simulink model "aileronAssembly"  (R2025a)
settings: Solver=VariableStepAuto  StartTime=0.0  StopTime=10.0  RelTol=1e-3
model workspace: external: MATLAB File aileronAssembly_DataFile.m (data not in the file)
undefined symbols (not defined in the file or in its folder): smiData, X, Y, Z
libraries: sm_lib x604, nesl_utility x1
(part 2 of 10)

== system aileronAssembly/Actuator_3/Cylinder_1_RIGID ==
  ReferenceFrame : sm_lib/Frames and Transforms/Reference Frame
  Solid : sm_lib/Body Elements/File Solid  ExtGeomFileName=Cylinder.step  UnitType=FromFile  ExtGeomFileUnits=m  StepReaderType=HEX  ExportConvexHullGeometry=off  InertiaType=Custom  BasedOnType=Density  Density=1000  DensityUnits=kg/m^3  Mass=smiData.Solid(7).mass  MassUnits=kg  CenterOfMass=smiData.Solid(7).CoM  CenterOfMassUnits=m  MomentsOfInertia=smiData.Solid(7).MoI  MomentsOfInertiaUnits=kg*m^2  ProductsOfInertia=smiData.Solid(7).PoI  ProductsOfInertiaUnits=kg*m^2  GraphicType=FromGeometry  MarkerShape=Sphere  MarkerSize=10  GraphicVisPropType=SimpleVisualProperties  GraphicDiffuseColor=smiData.Solid(7).color  GraphicOpacity=smiData.Solid(7).opacity  GraphicSpecularColor=[0.5 0.5 0.5 1.0]  GraphicAmbientColor=[0.15 0.15 0.15 1.0]  GraphicEmissiveColor=[0.0 0.0 0.0 1.0]  GraphicShininess=75  DoExposeReferenceFrame=on  SerializedFrames=<Frames/>
  Transform : sm_lib/Frames and Transforms/Rigid Transform  RotationMethod=ArbitraryAxis  FollAlignAxisA=+X  BaseAlignAxisA=+Y  FollAlignAxisB=+Y  BaseAlignAxisB=+Z  RotationStandardAxis=+Z  RotationAngle=smiData.RigidTransform(169).angle  RotationAngleUnits=rad  RotationArbitraryAxis=smiData.RigidTransform(169).axis  RotationSequenceAxes=FollowerAxes  RotationSequence=XYX  RotationSequenceAngles=[0 0 0]  RotationSequenceAnglesUnits=deg  RotationMatrix=[1 0 0; 0 1 0; 0 0 1]  Quaternion=[1 0 0 0]  TranslationMethod=Cartesian  TranslationCartesianOffset=smiData.RigidTransform(169).translation  TranslationCartesianOffsetUnits=m  TranslationStandardAxis=+Z  TranslationStandardOffset=0  TranslationStandardOffsetUnits=m  TranslationROffset=0  TranslationROffsetUnits=m  TranslationThetaOffset=0  TranslationThetaOffsetUnits=deg  TranslationZOffset=0  TranslationZOffsetUnits=m
  Transform1 : sm_lib/Frames and Transforms/Rigid Transform  RotationMethod=ArbitraryAxis  FollAlignAxisA=+X  BaseAlignAxisA=+Y  FollAlignAxisB=+Y  BaseAlignAxisB=+Z  RotationStandardAxis=+Z  RotationAngle=smiData.RigidTransform(196).angle  RotationAngleUnits=rad  RotationArbitraryAxis=smiData.RigidTransform(196).axis  RotationSequenceAxes=FollowerAxes  RotationSequence=XYX  RotationSequenceAngles=[0 0 0]  RotationSequenceAnglesUnits=deg  RotationMatrix=[1 0 0; 0 1 0; 0 0 1]  Quaternion=[1 0 0 0]  TranslationMethod=Cartesian  TranslationCartesianOffset=smiData.RigidTransform(196).translation  TranslationCartesianOffsetUnits=m  TranslationStandardAxis=+Z  TranslationStandardOffset=0  TranslationStandardOffsetUnits=m  TranslationROffset=0  TranslationROffsetUnits=m  TranslationThetaOffset=0  TranslationThetaOffsetUnits=deg  TranslationZOffset=0  TranslationZOffsetUnits=m
  F1 : PMIOPort  Side=Left
  F : PMIOPort  Port=2  Side=Right
  connections:
  Solid/RConn1 -- ReferenceFrame/RConn1 -- Transform/LConn1 -- Transform1/LConn1
  Transform/RConn1 -- F/RConn1
  Transform1/RConn1 -- F1/RConn1

== system aileronAssembly/Actuator_3/Piston_1_RIGID ==
  ReferenceFrame : sm_lib/Frames and Transforms/Reference Frame
  Solid : sm_lib/Body Elements/File Solid  ExtGeomFileName=Piston.step  UnitType=FromFile  ExtGeomFileUnits=m  StepReaderType=HEX  ExportConvexHullGeometry=off  InertiaType=Custom  BasedOnType=Density  Density=1000  DensityUnits=kg/m^3  Mass=smiData.Solid(8).mass  MassUnits=kg  CenterOfMass=smiData.Solid(8).CoM  CenterOfMassUnits=m  MomentsOfInertia=smiData.Solid(8).MoI  MomentsOfInertiaUnits=kg*m^2  ProductsOfInertia=smiData.Solid(8).PoI  ProductsOfInertiaUnits=kg*m^2  GraphicType=FromGeometry  MarkerShape=Sphere  MarkerSize=10  GraphicVisPropType=SimpleVisualProperties  GraphicDiffuseColor=smiData.Solid(8).color  GraphicOpacity=smiData.Solid(8).opacity  GraphicSpecularColor=[0.5 0.5 0.5 1.0]  GraphicAmbientColor=[0.15 0.15 0.15 1.0]  GraphicEmissiveColor=[0.0 0.0 0.0 1.0]  GraphicShininess=75  DoExposeReferenceFrame=on  SerializedFrames=<Frames/>
  Transform : sm_lib/Frames and Transforms/Rigid Transform  RotationMethod=ArbitraryAxis  FollAlignAxisA=+X  BaseAlignAxisA=+Y  FollAlignAxisB=+Y  BaseAlignAxisB=+Z  RotationStandardAxis=+Z  RotationAngle=smiData.RigidTransform(170).angle  RotationAngleUnits=rad  RotationArbitraryAxis=smiData.RigidTransform(170).axis  RotationSequenceAxes=FollowerAxes  RotationSequence=XYX  RotationSequenceAngles=[0 0 0]  RotationSequenceAnglesUnits=deg  RotationMatrix=[1 0 0; 0 1 0; 0 0 1]  Quaternion=[1 0 0 0]  TranslationMethod=Cartesian  TranslationCartesianOffset=smiData.RigidTransform(170).translation  TranslationCartesianOffsetUnits=m  TranslationStandardAxis=+Z  TranslationStandardOffset=0  TranslationStandardOffsetUnits=m  TranslationROffset=0  TranslationROffsetUnits=m  TranslationThetaOffset=0  TranslationThetaOffsetUnits=deg  TranslationZOffset=0  TranslationZOffsetUnits=m
  Transform1 : sm_lib/Frames and Transforms/Rigid Transform  RotationMethod=ArbitraryAxis  FollAlignAxisA=+X  BaseAlignAxisA=+Y  FollAlignAxisB=+Y  BaseAlignAxisB=+Z  RotationStandardAxis=+Z  RotationAngle=smiData.RigidTransform(201).angle  RotationAngleUnits=rad  RotationArbitraryAxis=smiData.RigidTransform(201).axis  RotationSequenceAxes=FollowerAxes  RotationSequence=XYX  RotationSequenceAngles=[0 0 0]  RotationSequenceAnglesUnits=deg  RotationMatrix=[1 0 0; 0 1 0; 0 0 1]  Quaternion=[1 0 0 0]  TranslationMethod=Cartesian  TranslationCartesianOffset=smiData.RigidTransform(201).translation  TranslationCartesianOffsetUnits=m  TranslationStandardAxis=+Z  TranslationStandardOffset=0  TranslationStandardOffsetUnits=m  TranslationROffset=0  TranslationROffsetUnits=m  TranslationThetaOffset=0  TranslationThetaOffsetUnits=deg  TranslationZOffset=0  TranslationZOffsetUnits=m
  F1 : PMIOPort  Side=Left
  F : PMIOPort  Port=2  Side=Left
  connections:
  Solid/RConn1 -- ReferenceFrame/RConn1 -- Transform/LConn1 -- Transform1/LConn1
  Transform/RConn1 -- F/RConn1
  Transform1/RConn1 -- F1/RConn1

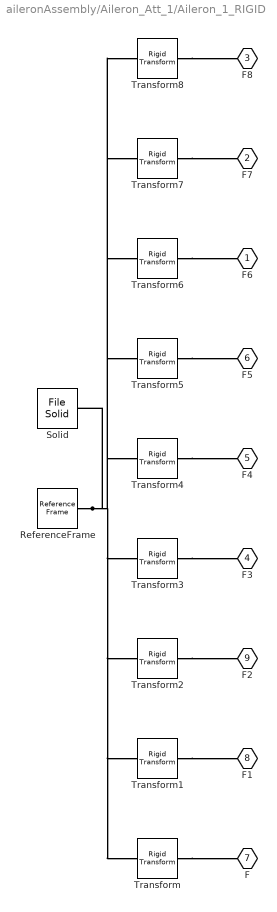
== system aileronAssembly/Aileron_Att_1/Aileron_1_RIGID ==
  ReferenceFrame : sm_lib/Frames and Transforms/Reference Frame
  Solid : sm_lib/Body Elements/File Solid  ExtGeomFileName=Aileron.step  UnitType=FromFile  ExtGeomFileUnits=m  StepReaderType=HEX  ExportConvexHullGeometry=off  InertiaType=Custom  BasedOnType=Density  Density=1000  DensityUnits=kg/m^3  Mass=smiData.Solid(9).mass  MassUnits=kg  CenterOfMass=smiData.Solid(9).CoM  CenterOfMassUnits=m  MomentsOfInertia=smiData.Solid(9).MoI  MomentsOfInertiaUnits=kg*m^2  ProductsOfInertia=smiData.Solid(9).PoI  ProductsOfInertiaUnits=kg*m^2  GraphicType=FromGeometry  MarkerShape=Sphere  MarkerSize=10  GraphicVisPropType=SimpleVisualProperties  GraphicDiffuseColor=smiData.Solid(9).color  GraphicOpacity=smiData.Solid(9).opacity  GraphicSpecularColor=[0.5 0.5 0.5 1.0]  GraphicAmbientColor=[0.15 0.15 0.15 1.0]  GraphicEmissiveColor=[0.0 0.0 0.0 1.0]  GraphicShininess=75  DoExposeReferenceFrame=on  SerializedFrames=<Frames/>
  Transform : sm_lib/Frames and Transforms/Rigid Transform  RotationMethod=ArbitraryAxis  FollAlignAxisA=+X  BaseAlignAxisA=+Y  FollAlignAxisB=+Y  BaseAlignAxisB=+Z  RotationStandardAxis=+Z  RotationAngle=smiData.RigidTransform(171).angle  RotationAngleUnits=rad  RotationArbitraryAxis=smiData.RigidTransform(171).axis  RotationSequenceAxes=FollowerAxes  RotationSequence=XYX  RotationSequenceAngles=[0 0 0]  RotationSequenceAnglesUnits=deg  RotationMatrix=[1 0 0; 0 1 0; 0 0 1]  Quaternion=[1 0 0 0]  TranslationMethod=Cartesian  TranslationCartesianOffset=smiData.RigidTransform(171).translation  TranslationCartesianOffsetUnits=m  TranslationStandardAxis=+Z  TranslationStandardOffset=0  TranslationStandardOffsetUnits=m  TranslationROffset=0  TranslationROffsetUnits=m  TranslationThetaOffset=0  TranslationThetaOffsetUnits=deg  TranslationZOffset=0  TranslationZOffsetUnits=m
  Transform1 : sm_lib/Frames and Transforms/Rigid Transform  RotationMethod=ArbitraryAxis  FollAlignAxisA=+X  BaseAlignAxisA=+Y  FollAlignAxisB=+Y  BaseAlignAxisB=+Z  RotationStandardAxis=+Z  RotationAngle=smiData.RigidTransform(173).angle  RotationAngleUnits=rad  RotationArbitraryAxis=smiData.RigidTransform(173).axis  RotationSequenceAxes=FollowerAxes  RotationSequence=XYX  RotationSequenceAngles=[0 0 0]  RotationSequenceAnglesUnits=deg  RotationMatrix=[1 0 0; 0 1 0; 0 0 1]  Quaternion=[1 0 0 0]  TranslationMethod=Cartesian  TranslationCartesianOffset=smiData.RigidTransform(173).translation  TranslationCartesianOffsetUnits=m  TranslationStandardAxis=+Z  TranslationStandardOffset=0  TranslationStandardOffsetUnits=m  TranslationROffset=0  TranslationROffsetUnits=m  TranslationThetaOffset=0  TranslationThetaOffsetUnits=deg  TranslationZOffset=0  TranslationZOffsetUnits=m
  Transform2 : sm_lib/Frames and Transforms/Rigid Transform  RotationMethod=ArbitraryAxis  FollAlignAxisA=+X  BaseAlignAxisA=+Y  FollAlignAxisB=+Y  BaseAlignAxisB=+Z  RotationStandardAxis=+Z  RotationAngle=smiData.RigidTransform(175).angle  RotationAngleUnits=rad  RotationArbitraryAxis=smiData.RigidTransform(175).axis  RotationSequenceAxes=FollowerAxes  RotationSequence=XYX  RotationSequenceAngles=[0 0 0]  RotationSequenceAnglesUnits=deg  RotationMatrix=[1 0 0; 0 1 0; 0 0 1]  Quaternion=[1 0 0 0]  TranslationMethod=Cartesian  TranslationCartesianOffset=smiData.RigidTransform(175).translation  TranslationCartesianOffsetUnits=m  TranslationStandardAxis=+Z  TranslationStandardOffset=0  TranslationStandardOffsetUnits=m  TranslationROffset=0  TranslationROffsetUnits=m  TranslationThetaOffset=0  TranslationThetaOffsetUnits=deg  TranslationZOffset=0  TranslationZOffsetUnits=m
  Transform3 : sm_lib/Frames and Transforms/Rigid Transform  RotationMethod=ArbitraryAxis  FollAlignAxisA=+X  BaseAlignAxisA=+Y  FollAlignAxisB=+Y  BaseAlignAxisB=+Z  RotationStandardAxis=+Z  RotationAngle=smiData.RigidTransform(177).angle  RotationAngleUnits=rad  RotationArbitraryAxis=smiData.RigidTransform(177).axis  RotationSequenceAxes=FollowerAxes  RotationSequence=XYX  RotationSequenceAngles=[0 0 0]  RotationSequenceAnglesUnits=deg  RotationMatrix=[1 0 0; 0 1 0; 0 0 1]  Quaternion=[1 0 0 0]  TranslationMethod=Cartesian  TranslationCartesianOffset=smiData.RigidTransform(177).translation  TranslationCartesianOffsetUnits=m  TranslationStandardAxis=+Z  TranslationStandardOffset=0  TranslationStandardOffsetUnits=m  TranslationROffset=0  TranslationROffsetUnits=m  TranslationThetaOffset=0  TranslationThetaOffsetUnits=deg  TranslationZOffset=0  TranslationZOffsetUnits=m
  Transform4 : sm_lib/Frames and Transforms/Rigid Transform  RotationMethod=ArbitraryAxis  FollAlignAxisA=+X  BaseAlignAxisA=+Y  FollAlignAxisB=+Y  BaseAlignAxisB=+Z  RotationStandardAxis=+Z  RotationAngle=smiData.RigidTransform(180).angle  RotationAngleUnits=rad  RotationArbitraryAxis=smiData.RigidTransform(180).axis  RotationSequenceAxes=FollowerAxes  RotationSequence=XYX  RotationSequenceAngles=[0 0 0]  RotationSequenceAnglesUnits=deg  RotationMatrix=[1 0 0; 0 1 0; 0 0 1]  Quaternion=[1 0 0 0]  TranslationMethod=Cartesian  TranslationCartesianOffset=smiData.RigidTransform(180).translation  TranslationCartesianOffsetUnits=m  TranslationStandardAxis=+Z  TranslationStandardOffset=0  TranslationStandardOffsetUnits=m  TranslationROffset=0  TranslationROffsetUnits=m  TranslationThetaOffset=0  TranslationThetaOffsetUnits=deg  TranslationZOffset=0  TranslationZOffsetUnits=m
  Transform5 : sm_lib/Frames and Transforms/Rigid Transform  RotationMethod=ArbitraryAxis  FollAlignAxisA=+X  BaseAlignAxisA=+Y  FollAlignAxisB=+Y  BaseAlignAxisB=+Z  RotationStandardAxis=+Z  RotationAngle=smiData.RigidTransform(182).angle  RotationAngleUnits=rad  RotationArbitraryAxis=smiData.RigidTransform(182).axis  RotationSequenceAxes=FollowerAxes  RotationSequence=XYX  RotationSequenceAngles=[0 0 0]  RotationSequenceAnglesUnits=deg  RotationMatrix=[1 0 0; 0 1 0; 0 0 1]  Quaternion=[1 0 0 0]  TranslationMethod=Cartesian  TranslationCartesianOffset=smiData.RigidTransform(182).translation  TranslationCartesianOffsetUnits=m  TranslationStandardAxis=+Z  TranslationStandardOffset=0  TranslationStandardOffsetUnits=m  TranslationROffset=0  TranslationROffsetUnits=m  TranslationThetaOffset=0  TranslationThetaOffsetUnits=deg  TranslationZOffset=0  TranslationZOffsetUnits=m
  Transform6 : sm_lib/Frames and Transforms/Rigid Transform  RotationMethod=ArbitraryAxis  FollAlignAxisA=+X  BaseAlignAxisA=+Y  FollAlignAxisB=+Y  BaseAlignAxisB=+Z  RotationStandardAxis=+Z  RotationAngle=smiData.RigidTransform(184).angle  RotationAngleUnits=rad  RotationArbitraryAxis=smiData.RigidTransform(184).axis  RotationSequenceAxes=FollowerAxes  RotationSequence=XYX  RotationSequenceAngles=[0 0 0]  RotationSequenceAnglesUnits=deg  RotationMatrix=[1 0 0; 0 1 0; 0 0 1]  Quaternion=[1 0 0 0]  TranslationMethod=Cartesian  TranslationCartesianOffset=smiData.RigidTransform(184).translation  TranslationCartesianOffsetUnits=m  TranslationStandardAxis=+Z  TranslationStandardOffset=0  TranslationStandardOffsetUnits=m  TranslationROffset=0  TranslationROffsetUnits=m  TranslationThetaOffset=0  TranslationThetaOffsetUnits=deg  TranslationZOffset=0  TranslationZOffsetUnits=m
  Transform7 : sm_lib/Frames and Transforms/Rigid Transform  RotationMethod=ArbitraryAxis  FollAlignAxisA=+X  BaseAlignAxisA=+Y  FollAlignAxisB=+Y  BaseAlignAxisB=+Z  RotationStandardAxis=+Z  RotationAngle=smiData.RigidTransform(186).angle  RotationAngleUnits=rad  RotationArbitraryAxis=smiData.RigidTransform(186).axis  RotationSequenceAxes=FollowerAxes  RotationSequence=XYX  RotationSequenceAngles=[0 0 0]  RotationSequenceAnglesUnits=deg  RotationMatrix=[1 0 0; 0 1 0; 0 0 1]  Quaternion=[1 0 0 0]  TranslationMethod=Cartesian  TranslationCartesianOffset=smiData.RigidTransform(186).translation  TranslationCartesianOffsetUnits=m  TranslationStandardAxis=+Z  TranslationStandardOffset=0  TranslationStandardOffsetUnits=m  TranslationROffset=0  TranslationROffsetUnits=m  TranslationThetaOffset=0  TranslationThetaOffsetUnits=deg  TranslationZOffset=0  TranslationZOffsetUnits=m
  Transform8 : sm_lib/Frames and Transforms/Rigid Transform  RotationMethod=ArbitraryAxis  FollAlignAxisA=+X  BaseAlignAxisA=+Y  FollAlignAxisB=+Y  BaseAlignAxisB=+Z  RotationStandardAxis=+Z  RotationAngle=smiData.RigidTransform(188).angle  RotationAngleUnits=rad  RotationArbitraryAxis=smiData.RigidTransform(188).axis  RotationSequenceAxes=FollowerAxes  RotationSequence=XYX  RotationSequenceAngles=[0 0 0]  RotationSequenceAnglesUnits=deg  RotationMatrix=[1 0 0; 0 1 0; 0 0 1]  Quaternion=[1 0 0 0]  TranslationMethod=Cartesian  TranslationCartesianOffset=smiData.RigidTransform(188).translation  TranslationCartesianOffsetUnits=m  TranslationStandardAxis=+Z  TranslationStandardOffset=0  TranslationStandardOffsetUnits=m  TranslationROffset=0  TranslationROffsetUnits=m  TranslationThetaOffset=0  TranslationThetaOffsetUnits=deg  TranslationZOffset=0  TranslationZOffsetUnits=m
  F6 : PMIOPort  Side=Left
  F7 : PMIOPort  Port=2  Side=Left
  F8 : PMIOPort  Port=3  Side=Left
  F3 : PMIOPort  Port=4  Side=Left
  F4 : PMIOPort  Port=5  Side=Left
  F5 : PMIOPort  Port=6  Side=Left
  F : PMIOPort  Port=7  Side=Left
  F1 : PMIOPort  Port=8  Side=Left
  F2 : PMIOPort  Port=9  Side=Left
  connections:
  Solid/RConn1 -- ReferenceFrame/RConn1 -- Transform/LConn1 -- Transform1/LConn1 -- Transform2/LConn1 -- Transform3/LConn1 -- Transform4/LConn1 -- Transform5/LConn1 -- Transform6/LConn1 -- Transform7/LConn1 -- Transform8/LConn1
  Transform/RConn1 -- F/RConn1
  Transform1/RConn1 -- F1/RConn1
  Transform2/RConn1 -- F2/RConn1
  Transform3/RConn1 -- F3/RConn1
  Transform4/RConn1 -- F4/RConn1
  Transform5/RConn1 -- F5/RConn1
  Transform6/RConn1 -- F6/RConn1
  Transform7/RConn1 -- F7/RConn1
  Transform8/RConn1 -- F8/RConn1

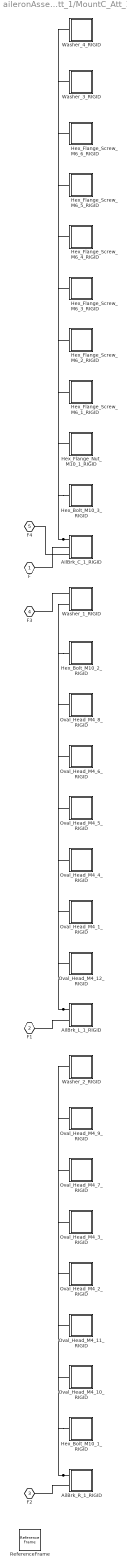
== system aileronAssembly/Aileron_Att_1/MountC_Att_1 ==
  AilBrk_C_1_RIGID : Subsystem
  AilBrk_L_1_RIGID : Subsystem
  AilBrk_R_1_RIGID : Subsystem
  Hex_Bolt_M10_1_RIGID : Subsystem
  Hex_Bolt_M10_2_RIGID : Subsystem
  Hex_Bolt_M10_3_RIGID : Subsystem
  Hex_Flange_Nut_M10_1_RIGID : Subsystem
  Hex_Flange_Screw_M6_1_RIGID : Subsystem
  Hex_Flange_Screw_M6_2_RIGID : Subsystem
  Hex_Flange_Screw_M6_3_RIGID : Subsystem
  Hex_Flange_Screw_M6_4_RIGID : Subsystem
  Hex_Flange_Screw_M6_5_RIGID : Subsystem
  Hex_Flange_Screw_M6_6_RIGID : Subsystem
  Oval_Head_M4_10_RIGID : Subsystem
  Oval_Head_M4_11_RIGID : Subsystem
  Oval_Head_M4_12_RIGID : Subsystem
  Oval_Head_M4_1_RIGID : Subsystem
  Oval_Head_M4_2_RIGID : Subsystem
  Oval_Head_M4_3_RIGID : Subsystem
  Oval_Head_M4_4_RIGID : Subsystem
  Oval_Head_M4_5_RIGID : Subsystem
  Oval_Head_M4_6_RIGID : Subsystem
  Oval_Head_M4_7_RIGID : Subsystem
  Oval_Head_M4_8_RIGID : Subsystem
  Oval_Head_M4_9_RIGID : Subsystem
  ReferenceFrame : sm_lib/Frames and Transforms/Reference Frame
  Washer_1_RIGID : Subsystem
  Washer_2_RIGID : Subsystem
  Washer_3_RIGID : Subsystem
  Washer_4_RIGID : Subsystem
  F : PMIOPort  Side=Left
  F1 : PMIOPort  Port=2  Side=Left
  F2 : PMIOPort  Port=3  Side=Left
  F3 : PMIOPort  Port=4  Side=Left
  F4 : PMIOPort  Port=5  Side=Left
  connections:
  Hex_Bolt_M10_1_RIGID/LConn1 -- AilBrk_R_1_RIGID/LConn1 -- Oval_Head_M4_10_RIGID/LConn1 -- Oval_Head_M4_11_RIGID/LConn1 -- Oval_Head_M4_2_RIGID/LConn1 -- Oval_Head_M4_3_RIGID/LConn1 -- Oval_Head_M4_7_RIGID/LConn1 -- Oval_Head_M4_9_RIGID/LConn1 -- Washer_2_RIGID/LConn1
  Hex_Bolt_M10_3_RIGID/LConn1 -- AilBrk_C_1_RIGID/LConn1 -- Hex_Flange_Nut_M10_1_RIGID/LConn1 -- Hex_Flange_Screw_M6_1_RIGID/LConn1 -- Hex_Flange_Screw_M6_2_RIGID/LConn1 -- Hex_Flange_Screw_M6_3_RIGID/LConn1 -- Hex_Flange_Screw_M6_4_RIGID/LConn1 -- Hex_Flange_Screw_M6_5_RIGID/LConn1 -- Hex_Flange_Screw_M6_6_RIGID/LConn1 -- Washer_3_RIGID/LConn1 -- Washer_4_RIGID/LConn1
  Hex_Bolt_M10_2_RIGID/LConn1 -- AilBrk_L_1_RIGID/LConn1 -- Oval_Head_M4_12_RIGID/LConn1 -- Oval_Head_M4_1_RIGID/LConn1 -- Oval_Head_M4_4_RIGID/LConn1 -- Oval_Head_M4_5_RIGID/LConn1 -- Oval_Head_M4_6_RIGID/LConn1 -- Oval_Head_M4_8_RIGID/LConn1 -- Washer_1_RIGID/LConn2
  AilBrk_C_1_RIGID/LConn2 -- F/RConn1
  AilBrk_L_1_RIGID/LConn2 -- F1/RConn1
  AilBrk_R_1_RIGID/LConn2 -- F2/RConn1
  Washer_1_RIGID/LConn1 -- F3/RConn1
  AilBrk_C_1_RIGID/LConn3 -- F4/RConn1

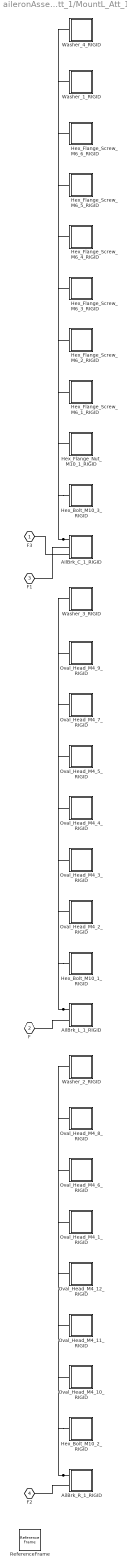
== system aileronAssembly/Aileron_Att_1/MountL_Att_1 ==
  AilBrk_C_1_RIGID : Subsystem
  AilBrk_L_1_RIGID : Subsystem
  AilBrk_R_1_RIGID : Subsystem
  Hex_Bolt_M10_1_RIGID : Subsystem
  Hex_Bolt_M10_2_RIGID : Subsystem
  Hex_Bolt_M10_3_RIGID : Subsystem
  Hex_Flange_Nut_M10_1_RIGID : Subsystem
  Hex_Flange_Screw_M6_1_RIGID : Subsystem
  Hex_Flange_Screw_M6_2_RIGID : Subsystem
  Hex_Flange_Screw_M6_3_RIGID : Subsystem
  Hex_Flange_Screw_M6_4_RIGID : Subsystem
  Hex_Flange_Screw_M6_5_RIGID : Subsystem
  Hex_Flange_Screw_M6_6_RIGID : Subsystem
  Oval_Head_M4_10_RIGID : Subsystem
  Oval_Head_M4_11_RIGID : Subsystem
  Oval_Head_M4_12_RIGID : Subsystem
  Oval_Head_M4_1_RIGID : Subsystem
  Oval_Head_M4_2_RIGID : Subsystem
  Oval_Head_M4_3_RIGID : Subsystem
  Oval_Head_M4_4_RIGID : Subsystem
  Oval_Head_M4_5_RIGID : Subsystem
  Oval_Head_M4_6_RIGID : Subsystem
  Oval_Head_M4_7_RIGID : Subsystem
  Oval_Head_M4_8_RIGID : Subsystem
  Oval_Head_M4_9_RIGID : Subsystem
  ReferenceFrame : sm_lib/Frames and Transforms/Reference Frame
  Washer_1_RIGID : Subsystem
  Washer_2_RIGID : Subsystem
  Washer_3_RIGID : Subsystem
  Washer_4_RIGID : Subsystem
  F3 : PMIOPort  Side=Left
  F : PMIOPort  Port=2  Side=Left
  F1 : PMIOPort  Port=3  Side=Left
  F2 : PMIOPort  Port=4  Side=Left
  connections:
  Hex_Bolt_M10_2_RIGID/LConn1 -- AilBrk_R_1_RIGID/LConn1 -- Oval_Head_M4_10_RIGID/LConn1 -- Oval_Head_M4_11_RIGID/LConn1 -- Oval_Head_M4_12_RIGID/LConn1 -- Oval_Head_M4_1_RIGID/LConn1 -- Oval_Head_M4_6_RIGID/LConn1 -- Oval_Head_M4_8_RIGID/LConn1 -- Washer_2_RIGID/LConn1
  Hex_Bolt_M10_1_RIGID/LConn1 -- AilBrk_L_1_RIGID/LConn1 -- Oval_Head_M4_2_RIGID/LConn1 -- Oval_Head_M4_3_RIGID/LConn1 -- Oval_Head_M4_4_RIGID/LConn1 -- Oval_Head_M4_5_RIGID/LConn1 -- Oval_Head_M4_7_RIGID/LConn1 -- Oval_Head_M4_9_RIGID/LConn1 -- Washer_3_RIGID/LConn1
  Hex_Bolt_M10_3_RIGID/LConn1 -- AilBrk_C_1_RIGID/LConn1 -- Hex_Flange_Nut_M10_1_RIGID/LConn1 -- Hex_Flange_Screw_M6_1_RIGID/LConn1 -- Hex_Flange_Screw_M6_2_RIGID/LConn1 -- Hex_Flange_Screw_M6_3_RIGID/LConn1 -- Hex_Flange_Screw_M6_4_RIGID/LConn1 -- Hex_Flange_Screw_M6_5_RIGID/LConn1 -- Hex_Flange_Screw_M6_6_RIGID/LConn1 -- Washer_1_RIGID/LConn1 -- Washer_4_RIGID/LConn1
  AilBrk_L_1_RIGID/LConn2 -- F/RConn1
  AilBrk_C_1_RIGID/LConn2 -- F1/RConn1
  AilBrk_R_1_RIGID/LConn2 -- F2/RConn1
  AilBrk_C_1_RIGID/LConn3 -- F3/RConn1

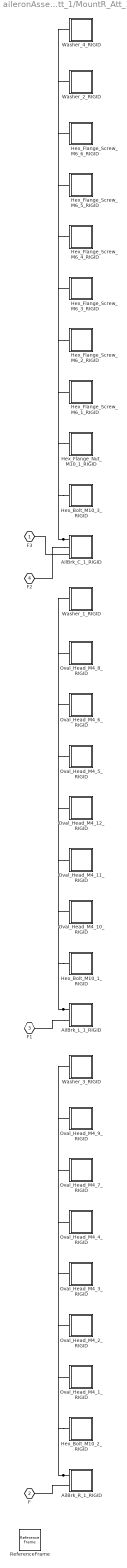
== system aileronAssembly/Aileron_Att_1/MountR_Att_1 ==
  AilBrk_C_1_RIGID : Subsystem
  AilBrk_L_1_RIGID : Subsystem
  AilBrk_R_1_RIGID : Subsystem
  Hex_Bolt_M10_1_RIGID : Subsystem
  Hex_Bolt_M10_2_RIGID : Subsystem
  Hex_Bolt_M10_3_RIGID : Subsystem
  Hex_Flange_Nut_M10_1_RIGID : Subsystem
  Hex_Flange_Screw_M6_1_RIGID : Subsystem
  Hex_Flange_Screw_M6_2_RIGID : Subsystem
  Hex_Flange_Screw_M6_3_RIGID : Subsystem
  Hex_Flange_Screw_M6_4_RIGID : Subsystem
  Hex_Flange_Screw_M6_5_RIGID : Subsystem
  Hex_Flange_Screw_M6_6_RIGID : Subsystem
  Oval_Head_M4_10_RIGID : Subsystem
  Oval_Head_M4_11_RIGID : Subsystem
  Oval_Head_M4_12_RIGID : Subsystem
  Oval_Head_M4_1_RIGID : Subsystem
  Oval_Head_M4_2_RIGID : Subsystem
  Oval_Head_M4_3_RIGID : Subsystem
  Oval_Head_M4_4_RIGID : Subsystem
  Oval_Head_M4_5_RIGID : Subsystem
  Oval_Head_M4_6_RIGID : Subsystem
  Oval_Head_M4_7_RIGID : Subsystem
  Oval_Head_M4_8_RIGID : Subsystem
  Oval_Head_M4_9_RIGID : Subsystem
  ReferenceFrame : sm_lib/Frames and Transforms/Reference Frame
  Washer_1_RIGID : Subsystem
  Washer_2_RIGID : Subsystem
  Washer_3_RIGID : Subsystem
  Washer_4_RIGID : Subsystem
  F3 : PMIOPort  Side=Left
  F : PMIOPort  Port=2  Side=Left
  F1 : PMIOPort  Port=3  Side=Left
  F2 : PMIOPort  Port=4  Side=Left
  connections:
  Hex_Bolt_M10_1_RIGID/LConn1 -- AilBrk_L_1_RIGID/LConn1 -- Oval_Head_M4_10_RIGID/LConn1 -- Oval_Head_M4_11_RIGID/LConn1 -- Oval_Head_M4_12_RIGID/LConn1 -- Oval_Head_M4_5_RIGID/LConn1 -- Oval_Head_M4_6_RIGID/LConn1 -- Oval_Head_M4_8_RIGID/LConn1 -- Washer_1_RIGID/LConn1
  Hex_Bolt_M10_2_RIGID/LConn1 -- AilBrk_R_1_RIGID/LConn1 -- Oval_Head_M4_1_RIGID/LConn1 -- Oval_Head_M4_2_RIGID/LConn1 -- Oval_Head_M4_3_RIGID/LConn1 -- Oval_Head_M4_4_RIGID/LConn1 -- Oval_Head_M4_7_RIGID/LConn1 -- Oval_Head_M4_9_RIGID/LConn1 -- Washer_3_RIGID/LConn1
  Hex_Bolt_M10_3_RIGID/LConn1 -- AilBrk_C_1_RIGID/LConn1 -- Hex_Flange_Nut_M10_1_RIGID/LConn1 -- Hex_Flange_Screw_M6_1_RIGID/LConn1 -- Hex_Flange_Screw_M6_2_RIGID/LConn1 -- Hex_Flange_Screw_M6_3_RIGID/LConn1 -- Hex_Flange_Screw_M6_4_RIGID/LConn1 -- Hex_Flange_Screw_M6_5_RIGID/LConn1 -- Hex_Flange_Screw_M6_6_RIGID/LConn1 -- Washer_2_RIGID/LConn1 -- Washer_4_RIGID/LConn1
  AilBrk_R_1_RIGID/LConn2 -- F/RConn1
  AilBrk_L_1_RIGID/LConn2 -- F1/RConn1
  AilBrk_C_1_RIGID/LConn2 -- F2/RConn1
  AilBrk_C_1_RIGID/LConn3 -- F3/RConn1

== system aileronAssembly/MountBrackets_1/MountC_1 ==
  Hex_Nut_M10_1_RIGID : Subsystem
  Hex_Screw_M10_1_RIGID : Subsystem
  Hex_Screw_M5_1_RIGID : Subsystem
  Hex_Screw_M5_2_RIGID : Subsystem
  Hex_Screw_M5_3_RIGID : Subsystem
  Hex_Screw_M5_4_RIGID : Subsystem
  Mount_1_RIGID : Subsystem
  Transform : sm_lib/Frames and Transforms/Rigid Transform  RotationMethod=ArbitraryAxis  FollAlignAxisA=+X  BaseAlignAxisA=+Y  FollAlignAxisB=+Y  BaseAlignAxisB=+Z  RotationStandardAxis=+Z  RotationAngle=smiData.RigidTransform(207).angle  RotationAngleUnits=rad  RotationArbitraryAxis=smiData.RigidTransform(207).axis  RotationSequenceAxes=FollowerAxes  RotationSequence=XYX  RotationSequenceAngles=[0 0 0]  RotationSequenceAnglesUnits=deg  RotationMatrix=[1 0 0; 0 1 0; 0 0 1]  Quaternion=[1 0 0 0]  TranslationMethod=Cartesian  TranslationCartesianOffset=smiData.RigidTransform(207).translation  TranslationCartesianOffsetUnits=m  TranslationStandardAxis=+Z  TranslationStandardOffset=0  TranslationStandardOffsetUnits=m  TranslationROffset=0  TranslationROffsetUnits=m  TranslationThetaOffset=0  TranslationThetaOffsetUnits=deg  TranslationZOffset=0  TranslationZOffsetUnits=m
  F : PMIOPort  Side=Left
  F1 : PMIOPort  Port=2  Side=Left
  connections:
  Hex_Screw_M10_1_RIGID/LConn1 -- Hex_Screw_M5_1_RIGID/LConn1 -- Mount_1_RIGID/LConn3 -- Hex_Nut_M10_1_RIGID/LConn1 -- Hex_Screw_M5_2_RIGID/LConn1 -- Hex_Screw_M5_3_RIGID/LConn1 -- Hex_Screw_M5_4_RIGID/LConn1
  Mount_1_RIGID/LConn2 -- F/RConn1
  Mount_1_RIGID/LConn1 -- Transform/RConn1
  F1/RConn1 -- Transform/LConn1

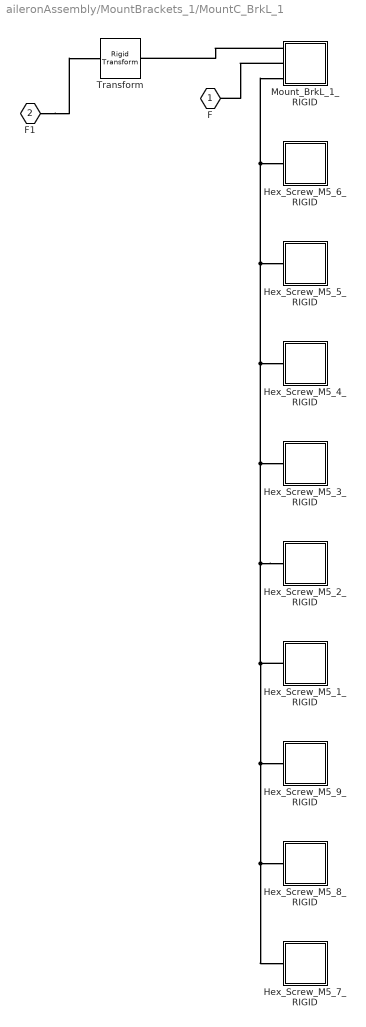
== system aileronAssembly/MountBrackets_1/MountC_BrkL_1 ==
  Hex_Screw_M5_1_RIGID : Subsystem
  Hex_Screw_M5_2_RIGID : Subsystem
  Hex_Screw_M5_3_RIGID : Subsystem
  Hex_Screw_M5_4_RIGID : Subsystem
  Hex_Screw_M5_5_RIGID : Subsystem
  Hex_Screw_M5_6_RIGID : Subsystem
  Hex_Screw_M5_7_RIGID : Subsystem
  Hex_Screw_M5_8_RIGID : Subsystem
  Hex_Screw_M5_9_RIGID : Subsystem
  Mount_BrkL_1_RIGID : Subsystem
  Transform : sm_lib/Frames and Transforms/Rigid Transform  RotationMethod=ArbitraryAxis  FollAlignAxisA=+X  BaseAlignAxisA=+Y  FollAlignAxisB=+Y  BaseAlignAxisB=+Z  RotationStandardAxis=+Z  RotationAngle=smiData.RigidTransform(209).angle  RotationAngleUnits=rad  RotationArbitraryAxis=smiData.RigidTransform(209).axis  RotationSequenceAxes=FollowerAxes  RotationSequence=XYX  RotationSequenceAngles=[0 0 0]  RotationSequenceAnglesUnits=deg  RotationMatrix=[1 0 0; 0 1 0; 0 0 1]  Quaternion=[1 0 0 0]  TranslationMethod=Cartesian  TranslationCartesianOffset=smiData.RigidTransform(209).translation  TranslationCartesianOffsetUnits=m  TranslationStandardAxis=+Z  TranslationStandardOffset=0  TranslationStandardOffsetUnits=m  TranslationROffset=0  TranslationROffsetUnits=m  TranslationThetaOffset=0  TranslationThetaOffsetUnits=deg  TranslationZOffset=0  TranslationZOffsetUnits=m
  F : PMIOPort  Side=Left
  F1 : PMIOPort  Port=2  Side=Left
  connections:
  Hex_Screw_M5_2_RIGID/LConn1 -- Hex_Screw_M5_6_RIGID/LConn1 -- Mount_BrkL_1_RIGID/LConn3 -- Hex_Screw_M5_5_RIGID/LConn1 -- Hex_Screw_M5_4_RIGID/LConn1 -- Hex_Screw_M5_3_RIGID/LConn1 -- Hex_Screw_M5_1_RIGID/LConn1 -- Hex_Screw_M5_7_RIGID/LConn1 -- Hex_Screw_M5_8_RIGID/LConn1 -- Hex_Screw_M5_9_RIGID/LConn1
  Mount_BrkL_1_RIGID/LConn2 -- F/RConn1
  Mount_BrkL_1_RIGID/LConn1 -- Transform/RConn1
  F1/RConn1 -- Transform/LConn1

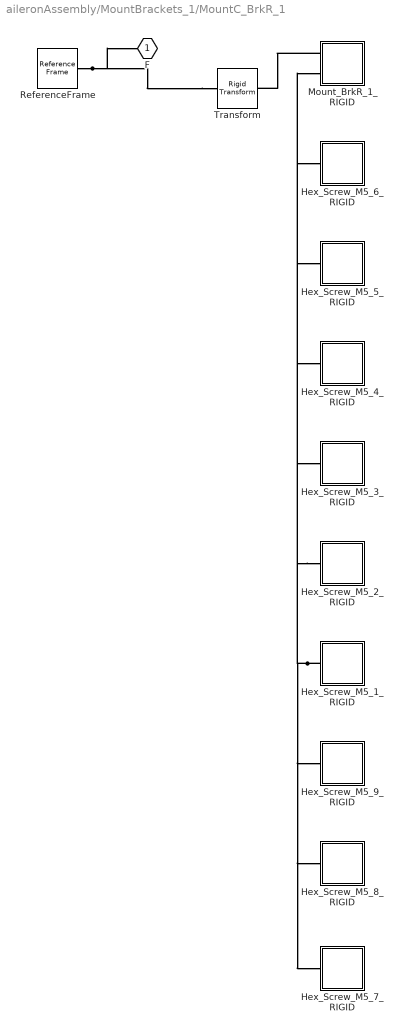
== system aileronAssembly/MountBrackets_1/MountC_BrkR_1 ==
  Hex_Screw_M5_1_RIGID : Subsystem
  Hex_Screw_M5_2_RIGID : Subsystem
  Hex_Screw_M5_3_RIGID : Subsystem
  Hex_Screw_M5_4_RIGID : Subsystem
  Hex_Screw_M5_5_RIGID : Subsystem
  Hex_Screw_M5_6_RIGID : Subsystem
  Hex_Screw_M5_7_RIGID : Subsystem
  Hex_Screw_M5_8_RIGID : Subsystem
  Hex_Screw_M5_9_RIGID : Subsystem
  Mount_BrkR_1_RIGID : Subsystem
  ReferenceFrame : sm_lib/Frames and Transforms/Reference Frame
  Transform : sm_lib/Frames and Transforms/Rigid Transform  RotationMethod=ArbitraryAxis  FollAlignAxisA=+X  BaseAlignAxisA=+Y  FollAlignAxisB=+Y  BaseAlignAxisB=+Z  RotationStandardAxis=+Z  RotationAngle=smiData.RigidTransform(204).angle  RotationAngleUnits=rad  RotationArbitraryAxis=smiData.RigidTransform(204).axis  RotationSequenceAxes=FollowerAxes  RotationSequence=XYX  RotationSequenceAngles=[0 0 0]  RotationSequenceAnglesUnits=deg  RotationMatrix=[1 0 0; 0 1 0; 0 0 1]  Quaternion=[1 0 0 0]  TranslationMethod=Cartesian  TranslationCartesianOffset=smiData.RigidTransform(204).translation  TranslationCartesianOffsetUnits=m  TranslationStandardAxis=+Z  TranslationStandardOffset=0  TranslationStandardOffsetUnits=m  TranslationROffset=0  TranslationROffsetUnits=m  TranslationThetaOffset=0  TranslationThetaOffsetUnits=deg  TranslationZOffset=0  TranslationZOffsetUnits=m
  F : PMIOPort  Side=Left
  connections:
  Hex_Screw_M5_2_RIGID/LConn1 -- Hex_Screw_M5_1_RIGID/LConn1 -- Hex_Screw_M5_3_RIGID/LConn1 -- Hex_Screw_M5_4_RIGID/LConn1 -- Hex_Screw_M5_5_RIGID/LConn1 -- Hex_Screw_M5_6_RIGID/LConn1 -- Hex_Screw_M5_7_RIGID/LConn1 -- Hex_Screw_M5_8_RIGID/LConn1 -- Hex_Screw_M5_9_RIGID/LConn1 -- Mount_BrkR_1_RIGID/LConn2
  Mount_BrkR_1_RIGID/LConn1 -- Transform/RConn1
  Transform/LConn1 -- ReferenceFrame/RConn1 -- F/RConn1

== system aileronAssembly/MountBrackets_1/MountL_1 ==
  Hex_Nut_M10_1_RIGID : Subsystem
  Hex_Screw_M10_1_RIGID : Subsystem
  Hex_Screw_M5_1_RIGID : Subsystem
  Hex_Screw_M5_2_RIGID : Subsystem
  Hex_Screw_M5_3_RIGID : Subsystem
  Hex_Screw_M5_4_RIGID : Subsystem
  Mount_1_RIGID : Subsystem
  Transform : sm_lib/Frames and Transforms/Rigid Transform  RotationMethod=ArbitraryAxis  FollAlignAxisA=+X  BaseAlignAxisA=+Y  FollAlignAxisB=+Y  BaseAlignAxisB=+Z  RotationStandardAxis=+Z  RotationAngle=smiData.RigidTransform(211).angle  RotationAngleUnits=rad  RotationArbitraryAxis=smiData.RigidTransform(211).axis  RotationSequenceAxes=FollowerAxes  RotationSequence=XYX  RotationSequenceAngles=[0 0 0]  RotationSequenceAnglesUnits=deg  RotationMatrix=[1 0 0; 0 1 0; 0 0 1]  Quaternion=[1 0 0 0]  TranslationMethod=Cartesian  TranslationCartesianOffset=smiData.RigidTransform(211).translation  TranslationCartesianOffsetUnits=m  TranslationStandardAxis=+Z  TranslationStandardOffset=0  TranslationStandardOffsetUnits=m  TranslationROffset=0  TranslationROffsetUnits=m  TranslationThetaOffset=0  TranslationThetaOffsetUnits=deg  TranslationZOffset=0  TranslationZOffsetUnits=m
  F : PMIOPort  Side=Left
  F1 : PMIOPort  Port=2  Side=Left
  connections:
  Hex_Screw_M10_1_RIGID/LConn1 -- Hex_Screw_M5_1_RIGID/LConn1 -- Mount_1_RIGID/LConn3 -- Hex_Nut_M10_1_RIGID/LConn1 -- Hex_Screw_M5_2_RIGID/LConn1 -- Hex_Screw_M5_3_RIGID/LConn1 -- Hex_Screw_M5_4_RIGID/LConn1
  Mount_1_RIGID/LConn2 -- F/RConn1
  Mount_1_RIGID/LConn1 -- Transform/RConn1
  F1/RConn1 -- Transform/LConn1

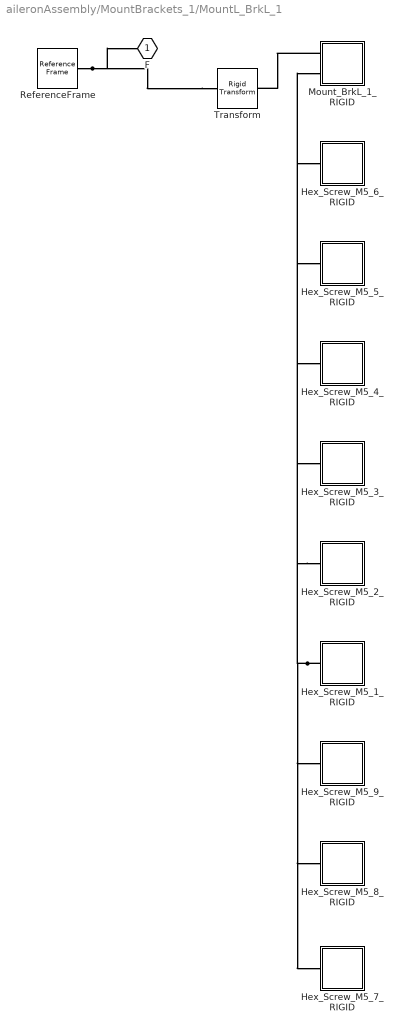
== system aileronAssembly/MountBrackets_1/MountL_BrkL_1 ==
  Hex_Screw_M5_1_RIGID : Subsystem
  Hex_Screw_M5_2_RIGID : Subsystem
  Hex_Screw_M5_3_RIGID : Subsystem
  Hex_Screw_M5_4_RIGID : Subsystem
  Hex_Screw_M5_5_RIGID : Subsystem
  Hex_Screw_M5_6_RIGID : Subsystem
  Hex_Screw_M5_7_RIGID : Subsystem
  Hex_Screw_M5_8_RIGID : Subsystem
  Hex_Screw_M5_9_RIGID : Subsystem
  Mount_BrkL_1_RIGID : Subsystem
  ReferenceFrame : sm_lib/Frames and Transforms/Reference Frame
  Transform : sm_lib/Frames and Transforms/Rigid Transform  RotationMethod=ArbitraryAxis  FollAlignAxisA=+X  BaseAlignAxisA=+Y  FollAlignAxisB=+Y  BaseAlignAxisB=+Z  RotationStandardAxis=+Z  RotationAngle=smiData.RigidTransform(203).angle  RotationAngleUnits=rad  RotationArbitraryAxis=smiData.RigidTransform(203).axis  RotationSequenceAxes=FollowerAxes  RotationSequence=XYX  RotationSequenceAngles=[0 0 0]  RotationSequenceAnglesUnits=deg  RotationMatrix=[1 0 0; 0 1 0; 0 0 1]  Quaternion=[1 0 0 0]  TranslationMethod=Cartesian  TranslationCartesianOffset=smiData.RigidTransform(203).translation  TranslationCartesianOffsetUnits=m  TranslationStandardAxis=+Z  TranslationStandardOffset=0  TranslationStandardOffsetUnits=m  TranslationROffset=0  TranslationROffsetUnits=m  TranslationThetaOffset=0  TranslationThetaOffsetUnits=deg  TranslationZOffset=0  TranslationZOffsetUnits=m
  F : PMIOPort  Side=Left
  connections:
  Hex_Screw_M5_2_RIGID/LConn1 -- Hex_Screw_M5_1_RIGID/LConn1 -- Hex_Screw_M5_3_RIGID/LConn1 -- Hex_Screw_M5_4_RIGID/LConn1 -- Hex_Screw_M5_5_RIGID/LConn1 -- Hex_Screw_M5_6_RIGID/LConn1 -- Hex_Screw_M5_7_RIGID/LConn1 -- Hex_Screw_M5_8_RIGID/LConn1 -- Hex_Screw_M5_9_RIGID/LConn1 -- Mount_BrkL_1_RIGID/LConn2
  Mount_BrkL_1_RIGID/LConn1 -- Transform/RConn1
  Transform/LConn1 -- ReferenceFrame/RConn1 -- F/RConn1

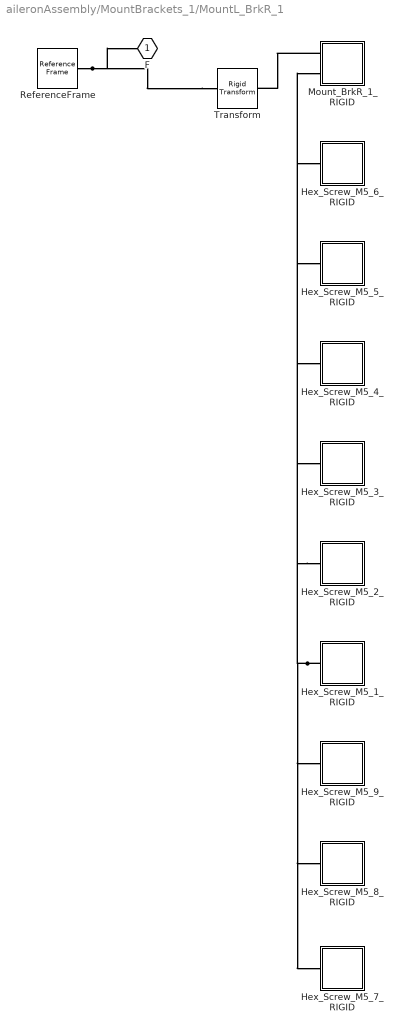
== system aileronAssembly/MountBrackets_1/MountL_BrkR_1 ==
  Hex_Screw_M5_1_RIGID : Subsystem
  Hex_Screw_M5_2_RIGID : Subsystem
  Hex_Screw_M5_3_RIGID : Subsystem
  Hex_Screw_M5_4_RIGID : Subsystem
  Hex_Screw_M5_5_RIGID : Subsystem
  Hex_Screw_M5_6_RIGID : Subsystem
  Hex_Screw_M5_7_RIGID : Subsystem
  Hex_Screw_M5_8_RIGID : Subsystem
  Hex_Screw_M5_9_RIGID : Subsystem
  Mount_BrkR_1_RIGID : Subsystem
  ReferenceFrame : sm_lib/Frames and Transforms/Reference Frame
  Transform : sm_lib/Frames and Transforms/Rigid Transform  RotationMethod=ArbitraryAxis  FollAlignAxisA=+X  BaseAlignAxisA=+Y  FollAlignAxisB=+Y  BaseAlignAxisB=+Z  RotationStandardAxis=+Z  RotationAngle=smiData.RigidTransform(208).angle  RotationAngleUnits=rad  RotationArbitraryAxis=smiData.RigidTransform(208).axis  RotationSequenceAxes=FollowerAxes  RotationSequence=XYX  RotationSequenceAngles=[0 0 0]  RotationSequenceAnglesUnits=deg  RotationMatrix=[1 0 0; 0 1 0; 0 0 1]  Quaternion=[1 0 0 0]  TranslationMethod=Cartesian  TranslationCartesianOffset=smiData.RigidTransform(208).translation  TranslationCartesianOffsetUnits=m  TranslationStandardAxis=+Z  TranslationStandardOffset=0  TranslationStandardOffsetUnits=m  TranslationROffset=0  TranslationROffsetUnits=m  TranslationThetaOffset=0  TranslationThetaOffsetUnits=deg  TranslationZOffset=0  TranslationZOffsetUnits=m
  F : PMIOPort  Side=Left
  connections:
  Hex_Screw_M5_2_RIGID/LConn1 -- Hex_Screw_M5_1_RIGID/LConn1 -- Hex_Screw_M5_3_RIGID/LConn1 -- Hex_Screw_M5_4_RIGID/LConn1 -- Hex_Screw_M5_5_RIGID/LConn1 -- Hex_Screw_M5_6_RIGID/LConn1 -- Hex_Screw_M5_7_RIGID/LConn1 -- Hex_Screw_M5_8_RIGID/LConn1 -- Hex_Screw_M5_9_RIGID/LConn1 -- Mount_BrkR_1_RIGID/LConn2
  Mount_BrkR_1_RIGID/LConn1 -- Transform/RConn1
  Transform/LConn1 -- ReferenceFrame/RConn1 -- F/RConn1

== system aileronAssembly/MountBrackets_1/MountR_1 ==
  Hex_Nut_M10_1_RIGID : Subsystem
  Hex_Screw_M10_1_RIGID : Subsystem
  Hex_Screw_M5_1_RIGID : Subsystem
  Hex_Screw_M5_2_RIGID : Subsystem
  Hex_Screw_M5_3_RIGID : Subsystem
  Hex_Screw_M5_4_RIGID : Subsystem
  Mount_1_RIGID : Subsystem
  SixDOF : sm_lib/Joints/Weld Joint  JointMode=Normal  CompositeWrenchDir=FollowerOnBase  CompositeWrenchFrame=BaseFrame  SenseConstraintForce=off  SenseConstraintTorque=off  SenseTotalForce=off  SenseTotalTorque=off
  Transform : sm_lib/Frames and Transforms/Rigid Transform  RotationMethod=ArbitraryAxis  FollAlignAxisA=+X  BaseAlignAxisA=+Y  FollAlignAxisB=+Y  BaseAlignAxisB=+Z  RotationStandardAxis=+Z  RotationAngle=smiData.RigidTransform(206).angle  RotationAngleUnits=rad  RotationArbitraryAxis=smiData.RigidTransform(206).axis  RotationSequenceAxes=FollowerAxes  RotationSequence=XYX  RotationSequenceAngles=[0 0 0]  RotationSequenceAnglesUnits=deg  RotationMatrix=[1 0 0; 0 1 0; 0 0 1]  Quaternion=[1 0 0 0]  TranslationMethod=Cartesian  TranslationCartesianOffset=smiData.RigidTransform(206).translation  TranslationCartesianOffsetUnits=m  TranslationStandardAxis=+Z  TranslationStandardOffset=0  TranslationStandardOffsetUnits=m  TranslationROffset=0  TranslationROffsetUnits=m  TranslationThetaOffset=0  TranslationThetaOffsetUnits=deg  TranslationZOffset=0  TranslationZOffsetUnits=m
  Transform1 : sm_lib/Frames and Transforms/Rigid Transform  RotationMethod=ArbitraryAxis  FollAlignAxisA=+X  BaseAlignAxisA=+Y  FollAlignAxisB=+Y  BaseAlignAxisB=+Z  RotationStandardAxis=+Z  RotationAngle=smiData.RigidTransform(218).angle  RotationAngleUnits=rad  RotationArbitraryAxis=smiData.RigidTransform(218).axis  RotationSequenceAxes=FollowerAxes  RotationSequence=XYX  RotationSequenceAngles=[0 0 0]  RotationSequenceAnglesUnits=deg  RotationMatrix=[1 0 0; 0 1 0; 0 0 1]  Quaternion=[1 0 0 0]  TranslationMethod=Cartesian  TranslationCartesianOffset=smiData.RigidTransform(218).translation  TranslationCartesianOffsetUnits=m  TranslationStandardAxis=+Z  TranslationStandardOffset=0  TranslationStandardOffsetUnits=m  TranslationROffset=0  TranslationROffsetUnits=m  TranslationThetaOffset=0  TranslationThetaOffsetUnits=deg  TranslationZOffset=0  TranslationZOffsetUnits=m
  F : PMIOPort  Side=Left
  F1 : PMIOPort  Port=2  Side=Left
  connections:
  Hex_Screw_M10_1_RIGID/LConn1 -- Hex_Nut_M10_1_RIGID/LConn1 -- Mount_1_RIGID/LConn3 -- Hex_Screw_M5_4_RIGID/LConn1 -- Hex_Screw_M5_2_RIGID/LConn1 -- Hex_Screw_M5_3_RIGID/LConn1 -- Hex_Screw_M5_1_RIGID/LConn1
  Mount_1_RIGID/LConn1 -- F/RConn1
  Mount_1_RIGID/LConn2 -- Transform/RConn1
  Transform1/LConn1 -- F1/RConn1 -- Transform/LConn1
  Hex_Screw_M5_3_RIGID/LConn2 -- SixDOF/RConn1
  SixDOF/LConn1 -- Transform1/RConn1

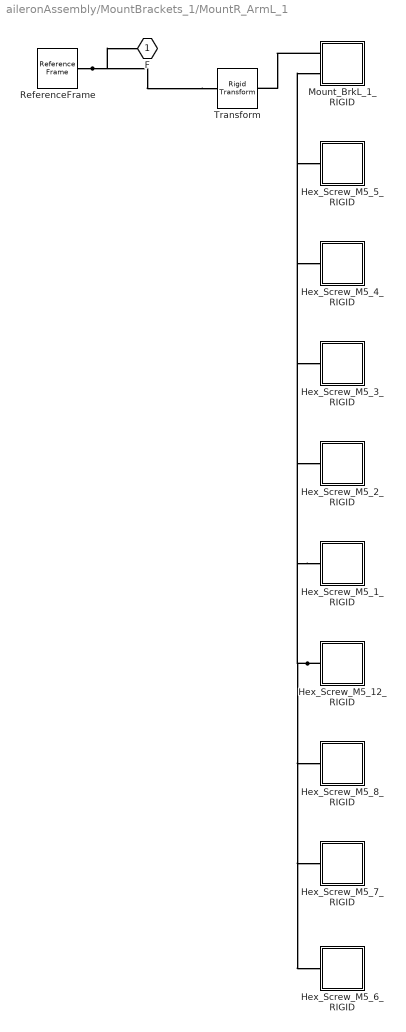
== system aileronAssembly/MountBrackets_1/MountR_ArmL_1 ==
  Hex_Screw_M5_12_RIGID : Subsystem
  Hex_Screw_M5_1_RIGID : Subsystem
  Hex_Screw_M5_2_RIGID : Subsystem
  Hex_Screw_M5_3_RIGID : Subsystem
  Hex_Screw_M5_4_RIGID : Subsystem
  Hex_Screw_M5_5_RIGID : Subsystem
  Hex_Screw_M5_6_RIGID : Subsystem
  Hex_Screw_M5_7_RIGID : Subsystem
  Hex_Screw_M5_8_RIGID : Subsystem
  Mount_BrkL_1_RIGID : Subsystem
  ReferenceFrame : sm_lib/Frames and Transforms/Reference Frame
  Transform : sm_lib/Frames and Transforms/Rigid Transform  RotationMethod=ArbitraryAxis  FollAlignAxisA=+X  BaseAlignAxisA=+Y  FollAlignAxisB=+Y  BaseAlignAxisB=+Z  RotationStandardAxis=+Z  RotationAngle=smiData.RigidTransform(210).angle  RotationAngleUnits=rad  RotationArbitraryAxis=smiData.RigidTransform(210).axis  RotationSequenceAxes=FollowerAxes  RotationSequence=XYX  RotationSequenceAngles=[0 0 0]  RotationSequenceAnglesUnits=deg  RotationMatrix=[1 0 0; 0 1 0; 0 0 1]  Quaternion=[1 0 0 0]  TranslationMethod=Cartesian  TranslationCartesianOffset=smiData.RigidTransform(210).translation  TranslationCartesianOffsetUnits=m  TranslationStandardAxis=+Z  TranslationStandardOffset=0  TranslationStandardOffsetUnits=m  TranslationROffset=0  TranslationROffsetUnits=m  TranslationThetaOffset=0  TranslationThetaOffsetUnits=deg  TranslationZOffset=0  TranslationZOffsetUnits=m
  F : PMIOPort  Side=Left
  connections:
  Hex_Screw_M5_1_RIGID/LConn1 -- Hex_Screw_M5_12_RIGID/LConn1 -- Hex_Screw_M5_2_RIGID/LConn1 -- Hex_Screw_M5_3_RIGID/LConn1 -- Hex_Screw_M5_4_RIGID/LConn1 -- Hex_Screw_M5_5_RIGID/LConn1 -- Hex_Screw_M5_6_RIGID/LConn1 -- Hex_Screw_M5_7_RIGID/LConn1 -- Hex_Screw_M5_8_RIGID/LConn1 -- Mount_BrkL_1_RIGID/LConn2
  Mount_BrkL_1_RIGID/LConn1 -- Transform/RConn1
  Transform/LConn1 -- ReferenceFrame/RConn1 -- F/RConn1

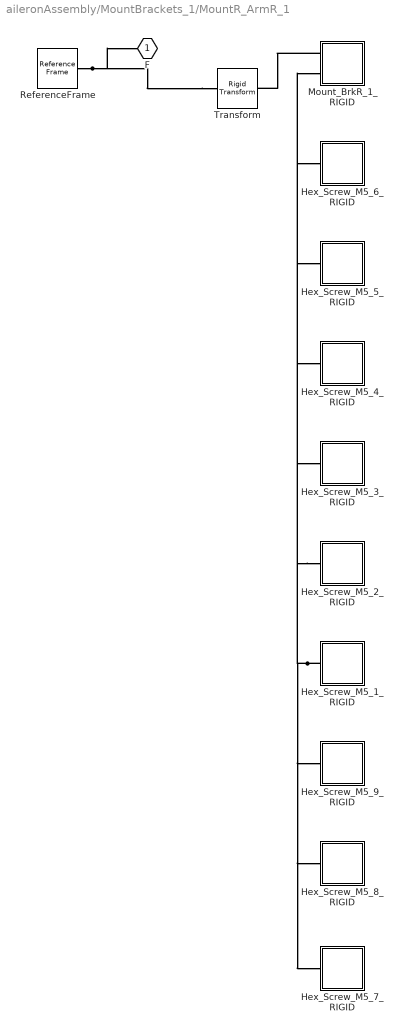
== system aileronAssembly/MountBrackets_1/MountR_ArmR_1 ==
  Hex_Screw_M5_1_RIGID : Subsystem
  Hex_Screw_M5_2_RIGID : Subsystem
  Hex_Screw_M5_3_RIGID : Subsystem
  Hex_Screw_M5_4_RIGID : Subsystem
  Hex_Screw_M5_5_RIGID : Subsystem
  Hex_Screw_M5_6_RIGID : Subsystem
  Hex_Screw_M5_7_RIGID : Subsystem
  Hex_Screw_M5_8_RIGID : Subsystem
  Hex_Screw_M5_9_RIGID : Subsystem
  Mount_BrkR_1_RIGID : Subsystem
  ReferenceFrame : sm_lib/Frames and Transforms/Reference Frame
  Transform : sm_lib/Frames and Transforms/Rigid Transform  RotationMethod=ArbitraryAxis  FollAlignAxisA=+X  BaseAlignAxisA=+Y  FollAlignAxisB=+Y  BaseAlignAxisB=+Z  RotationStandardAxis=+Z  RotationAngle=smiData.RigidTransform(205).angle  RotationAngleUnits=rad  RotationArbitraryAxis=smiData.RigidTransform(205).axis  RotationSequenceAxes=FollowerAxes  RotationSequence=XYX  RotationSequenceAngles=[0 0 0]  RotationSequenceAnglesUnits=deg  RotationMatrix=[1 0 0; 0 1 0; 0 0 1]  Quaternion=[1 0 0 0]  TranslationMethod=Cartesian  TranslationCartesianOffset=smiData.RigidTransform(205).translation  TranslationCartesianOffsetUnits=m  TranslationStandardAxis=+Z  TranslationStandardOffset=0  TranslationStandardOffsetUnits=m  TranslationROffset=0  TranslationROffsetUnits=m  TranslationThetaOffset=0  TranslationThetaOffsetUnits=deg  TranslationZOffset=0  TranslationZOffsetUnits=m
  F : PMIOPort  Side=Left
  connections:
  Hex_Screw_M5_2_RIGID/LConn1 -- Hex_Screw_M5_1_RIGID/LConn1 -- Hex_Screw_M5_3_RIGID/LConn1 -- Hex_Screw_M5_4_RIGID/LConn1 -- Hex_Screw_M5_5_RIGID/LConn1 -- Hex_Screw_M5_6_RIGID/LConn1 -- Hex_Screw_M5_7_RIGID/LConn1 -- Hex_Screw_M5_8_RIGID/LConn1 -- Hex_Screw_M5_9_RIGID/LConn1 -- Mount_BrkR_1_RIGID/LConn2
  Mount_BrkR_1_RIGID/LConn1 -- Transform/RConn1
  Transform/LConn1 -- ReferenceFrame/RConn1 -- F/RConn1

== system aileronAssembly/Aileron_Att_1/MountC_Att_1/AilBrk_C_1_RIGID ==
  ReferenceFrame : sm_lib/Frames and Transforms/Reference Frame
  Solid : sm_lib/Body Elements/File Solid  ExtGeomFileName=AilBrk_C.step  UnitType=FromFile  ExtGeomFileUnits=m  StepReaderType=HEX  ExportConvexHullGeometry=off  InertiaType=Custom  BasedOnType=Density  Density=1000  DensityUnits=kg/m^3  Mass=smiData.Solid(15).mass  MassUnits=kg  CenterOfMass=smiData.Solid(15).CoM  CenterOfMassUnits=m  MomentsOfInertia=smiData.Solid(15).MoI  MomentsOfInertiaUnits=kg*m^2  ProductsOfInertia=smiData.Solid(15).PoI  ProductsOfInertiaUnits=kg*m^2  GraphicType=FromGeometry  MarkerShape=Sphere  MarkerSize=10  GraphicVisPropType=SimpleVisualProperties  GraphicDiffuseColor=smiData.Solid(15).color  GraphicOpacity=smiData.Solid(15).opacity  GraphicSpecularColor=[0.5 0.5 0.5 1.0]  GraphicAmbientColor=[0.15 0.15 0.15 1.0]  GraphicEmissiveColor=[0.0 0.0 0.0 1.0]  GraphicShininess=75  DoExposeReferenceFrame=on  SerializedFrames=<Frames/>
  Transform : sm_lib/Frames and Transforms/Rigid Transform  RotationMethod=ArbitraryAxis  FollAlignAxisA=+X  BaseAlignAxisA=+Y  FollAlignAxisB=+Y  BaseAlignAxisB=+Z  RotationStandardAxis=+Z  RotationAngle=smiData.RigidTransform(98).angle  RotationAngleUnits=rad  RotationArbitraryAxis=smiData.RigidTransform(98).axis  RotationSequenceAxes=FollowerAxes  RotationSequence=XYX  RotationSequenceAngles=[0 0 0]  RotationSequenceAnglesUnits=deg  RotationMatrix=[1 0 0; 0 1 0; 0 0 1]  Quaternion=[1 0 0 0]  TranslationMethod=Cartesian  TranslationCartesianOffset=smiData.RigidTransform(98).translation  TranslationCartesianOffsetUnits=m  TranslationStandardAxis=+Z  TranslationStandardOffset=0  TranslationStandardOffsetUnits=m  TranslationROffset=0  TranslationROffsetUnits=m  TranslationThetaOffset=0  TranslationThetaOffsetUnits=deg  TranslationZOffset=0  TranslationZOffsetUnits=m
  Transform1 : sm_lib/Frames and Transforms/Rigid Transform  RotationMethod=ArbitraryAxis  FollAlignAxisA=+X  BaseAlignAxisA=+Y  FollAlignAxisB=+Y  BaseAlignAxisB=+Z  RotationStandardAxis=+Z  RotationAngle=smiData.RigidTransform(172).angle  RotationAngleUnits=rad  RotationArbitraryAxis=smiData.RigidTransform(172).axis  RotationSequenceAxes=FollowerAxes  RotationSequence=XYX  RotationSequenceAngles=[0 0 0]  RotationSequenceAnglesUnits=deg  RotationMatrix=[1 0 0; 0 1 0; 0 0 1]  Quaternion=[1 0 0 0]  TranslationMethod=Cartesian  TranslationCartesianOffset=smiData.RigidTransform(172).translation  TranslationCartesianOffsetUnits=m  TranslationStandardAxis=+Z  TranslationStandardOffset=0  TranslationStandardOffsetUnits=m  TranslationROffset=0  TranslationROffsetUnits=m  TranslationThetaOffset=0  TranslationThetaOffsetUnits=deg  TranslationZOffset=0  TranslationZOffsetUnits=m
  Transform2 : sm_lib/Frames and Transforms/Rigid Transform  RotationMethod=ArbitraryAxis  FollAlignAxisA=+X  BaseAlignAxisA=+Y  FollAlignAxisB=+Y  BaseAlignAxisB=+Z  RotationStandardAxis=+Z  RotationAngle=smiData.RigidTransform(200).angle  RotationAngleUnits=rad  RotationArbitraryAxis=smiData.RigidTransform(200).axis  RotationSequenceAxes=FollowerAxes  RotationSequence=XYX  RotationSequenceAngles=[0 0 0]  RotationSequenceAnglesUnits=deg  RotationMatrix=[1 0 0; 0 1 0; 0 0 1]  Quaternion=[1 0 0 0]  TranslationMethod=Cartesian  TranslationCartesianOffset=smiData.RigidTransform(200).translation  TranslationCartesianOffsetUnits=m  TranslationStandardAxis=+Z  TranslationStandardOffset=0  TranslationStandardOffsetUnits=m  TranslationROffset=0  TranslationROffsetUnits=m  TranslationThetaOffset=0  TranslationThetaOffsetUnits=deg  TranslationZOffset=0  TranslationZOffsetUnits=m
  G : PMIOPort  Side=Left
  F : PMIOPort  Port=2  Side=Left
  F1 : PMIOPort  Port=3  Side=Left
  connections:
  Solid/RConn1 -- ReferenceFrame/RConn1 -- Transform/RConn1 -- Transform1/LConn1 -- Transform2/LConn1
  Transform/LConn1 -- G/RConn1
  Transform1/RConn1 -- F/RConn1
  Transform2/RConn1 -- F1/RConn1

== system aileronAssembly/Aileron_Att_1/MountC_Att_1/AilBrk_L_1_RIGID ==
  ReferenceFrame : sm_lib/Frames and Transforms/Reference Frame
  Solid : sm_lib/Body Elements/File Solid  ExtGeomFileName=AilBrk_L.step  UnitType=FromFile  ExtGeomFileUnits=m  StepReaderType=HEX  ExportConvexHullGeometry=off  InertiaType=Custom  BasedOnType=Density  Density=1000  DensityUnits=kg/m^3  Mass=smiData.Solid(13).mass  MassUnits=kg  CenterOfMass=smiData.Solid(13).CoM  CenterOfMassUnits=m  MomentsOfInertia=smiData.Solid(13).MoI  MomentsOfInertiaUnits=kg*m^2  ProductsOfInertia=smiData.Solid(13).PoI  ProductsOfInertiaUnits=kg*m^2  GraphicType=FromGeometry  MarkerShape=Sphere  MarkerSize=10  GraphicVisPropType=SimpleVisualProperties  GraphicDiffuseColor=smiData.Solid(13).color  GraphicOpacity=smiData.Solid(13).opacity  GraphicSpecularColor=[0.5 0.5 0.5 1.0]  GraphicAmbientColor=[0.15 0.15 0.15 1.0]  GraphicEmissiveColor=[0.0 0.0 0.0 1.0]  GraphicShininess=75  DoExposeReferenceFrame=on  SerializedFrames=<Frames/>
  Transform : sm_lib/Frames and Transforms/Rigid Transform  RotationMethod=ArbitraryAxis  FollAlignAxisA=+X  BaseAlignAxisA=+Y  FollAlignAxisB=+Y  BaseAlignAxisB=+Z  RotationStandardAxis=+Z  RotationAngle=smiData.RigidTransform(103).angle  RotationAngleUnits=rad  RotationArbitraryAxis=smiData.RigidTransform(103).axis  RotationSequenceAxes=FollowerAxes  RotationSequence=XYX  RotationSequenceAngles=[0 0 0]  RotationSequenceAnglesUnits=deg  RotationMatrix=[1 0 0; 0 1 0; 0 0 1]  Quaternion=[1 0 0 0]  TranslationMethod=Cartesian  TranslationCartesianOffset=smiData.RigidTransform(103).translation  TranslationCartesianOffsetUnits=m  TranslationStandardAxis=+Z  TranslationStandardOffset=0  TranslationStandardOffsetUnits=m  TranslationROffset=0  TranslationROffsetUnits=m  TranslationThetaOffset=0  TranslationThetaOffsetUnits=deg  TranslationZOffset=0  TranslationZOffsetUnits=m
  Transform1 : sm_lib/Frames and Transforms/Rigid Transform  RotationMethod=ArbitraryAxis  FollAlignAxisA=+X  BaseAlignAxisA=+Y  FollAlignAxisB=+Y  BaseAlignAxisB=+Z  RotationStandardAxis=+Z  RotationAngle=smiData.RigidTransform(174).angle  RotationAngleUnits=rad  RotationArbitraryAxis=smiData.RigidTransform(174).axis  RotationSequenceAxes=FollowerAxes  RotationSequence=XYX  RotationSequenceAngles=[0 0 0]  RotationSequenceAnglesUnits=deg  RotationMatrix=[1 0 0; 0 1 0; 0 0 1]  Quaternion=[1 0 0 0]  TranslationMethod=Cartesian  TranslationCartesianOffset=smiData.RigidTransform(174).translation  TranslationCartesianOffsetUnits=m  TranslationStandardAxis=+Z  TranslationStandardOffset=0  TranslationStandardOffsetUnits=m  TranslationROffset=0  TranslationROffsetUnits=m  TranslationThetaOffset=0  TranslationThetaOffsetUnits=deg  TranslationZOffset=0  TranslationZOffsetUnits=m
  G : PMIOPort  Side=Left
  F : PMIOPort  Port=2  Side=Left
  connections:
  Solid/RConn1 -- ReferenceFrame/RConn1 -- Transform/RConn1 -- Transform1/LConn1
  Transform/LConn1 -- G/RConn1
  Transform1/RConn1 -- F/RConn1

== system aileronAssembly/Aileron_Att_1/MountC_Att_1/AilBrk_R_1_RIGID ==
  ReferenceFrame : sm_lib/Frames and Transforms/Reference Frame
  Solid : sm_lib/Body Elements/File Solid  ExtGeomFileName=AilBrk_R.step  UnitType=FromFile  ExtGeomFileUnits=m  StepReaderType=HEX  ExportConvexHullGeometry=off  InertiaType=Custom  BasedOnType=Density  Density=1000  DensityUnits=kg/m^3  Mass=smiData.Solid(16).mass  MassUnits=kg  CenterOfMass=smiData.Solid(16).CoM  CenterOfMassUnits=m  MomentsOfInertia=smiData.Solid(16).MoI  MomentsOfInertiaUnits=kg*m^2  ProductsOfInertia=smiData.Solid(16).PoI  ProductsOfInertiaUnits=kg*m^2  GraphicType=FromGeometry  MarkerShape=Sphere  MarkerSize=10  GraphicVisPropType=SimpleVisualProperties  GraphicDiffuseColor=smiData.Solid(16).color  GraphicOpacity=smiData.Solid(16).opacity  GraphicSpecularColor=[0.5 0.5 0.5 1.0]  GraphicAmbientColor=[0.15 0.15 0.15 1.0]  GraphicEmissiveColor=[0.0 0.0 0.0 1.0]  GraphicShininess=75  DoExposeReferenceFrame=on  SerializedFrames=<Frames/>
  Transform : sm_lib/Frames and Transforms/Rigid Transform  RotationMethod=ArbitraryAxis  FollAlignAxisA=+X  BaseAlignAxisA=+Y  FollAlignAxisB=+Y  BaseAlignAxisB=+Z  RotationStandardAxis=+Z  RotationAngle=smiData.RigidTransform(82).angle  RotationAngleUnits=rad  RotationArbitraryAxis=smiData.RigidTransform(82).axis  RotationSequenceAxes=FollowerAxes  RotationSequence=XYX  RotationSequenceAngles=[0 0 0]  RotationSequenceAnglesUnits=deg  RotationMatrix=[1 0 0; 0 1 0; 0 0 1]  Quaternion=[1 0 0 0]  TranslationMethod=Cartesian  TranslationCartesianOffset=smiData.RigidTransform(82).translation  TranslationCartesianOffsetUnits=m  TranslationStandardAxis=+Z  TranslationStandardOffset=0  TranslationStandardOffsetUnits=m  TranslationROffset=0  TranslationROffsetUnits=m  TranslationThetaOffset=0  TranslationThetaOffsetUnits=deg  TranslationZOffset=0  TranslationZOffsetUnits=m
  Transform1 : sm_lib/Frames and Transforms/Rigid Transform  RotationMethod=ArbitraryAxis  FollAlignAxisA=+X  BaseAlignAxisA=+Y  FollAlignAxisB=+Y  BaseAlignAxisB=+Z  RotationStandardAxis=+Z  RotationAngle=smiData.RigidTransform(176).angle  RotationAngleUnits=rad  RotationArbitraryAxis=smiData.RigidTransform(176).axis  RotationSequenceAxes=FollowerAxes  RotationSequence=XYX  RotationSequenceAngles=[0 0 0]  RotationSequenceAnglesUnits=deg  RotationMatrix=[1 0 0; 0 1 0; 0 0 1]  Quaternion=[1 0 0 0]  TranslationMethod=Cartesian  TranslationCartesianOffset=smiData.RigidTransform(176).translation  TranslationCartesianOffsetUnits=m  TranslationStandardAxis=+Z  TranslationStandardOffset=0  TranslationStandardOffsetUnits=m  TranslationROffset=0  TranslationROffsetUnits=m  TranslationThetaOffset=0  TranslationThetaOffsetUnits=deg  TranslationZOffset=0  TranslationZOffsetUnits=m
  G : PMIOPort  Side=Left
  F : PMIOPort  Port=2  Side=Left
  connections:
  Solid/RConn1 -- ReferenceFrame/RConn1 -- Transform/RConn1 -- Transform1/LConn1
  Transform/LConn1 -- G/RConn1
  Transform1/RConn1 -- F/RConn1
